simulink model "ZeroForceDrag_ThreeJoints"  (R2018b)
settings: Solver=FixedStepDiscrete  StartTime=0.0  StopTime=Inf  FixedStep=0.001  RelTol=1e-3  EnableMultiTasking=on
PreLoadFcn:
  | clear,clc;
undefined symbols (not defined in the file): J1, J2, J3, J4, J5, J6, J7, Motor_Current, Motor_Position, Motor_Velocity, Send_GUIdata
libraries: c280xlib x14, simulink x5, idelinklib_common x1
(part 4 of 4)

== stateflow chart ZeroForceDrag_ThreeJoints/DynamicCalculation/DriveMotor/驱动器指令/Chart2 ==
  state bx = check(write) [function]
  state MSG = UM1 [function]
  state start = start_arm(StartRobot) [function]
  state State05
    entry:
    start=0;
    during:
    start=start_arm(StartRobot);
    %启动机械臂
  state State01
    entry:
    bx=0;
    during:
    bx=check(write);
  state State06
    entry:
    MSG = UM1;
  state State03
    entry:
    MSG = BG;
  state MSG = TF(Current) [function]
  state State04
    entry:
    during:
    MSG = TF(Current);
  state MSG = BG [function]
  State01 -> State06 : [bx>0]
  (default) -> State05
  State05 -> State01 : [start>0]
  State06 -> State03
  State03 -> State04
  data: write function_input uint16 size=1; bx function_output uint16 size=1; MSG function_output; StartRobot function_input uint16 size=1; start function_output uint16 size=1; MSG function_output; Current function_input uint16 size=[1 6]; MSG function_output; MSG output; Current input size=[1 6]; write input uint16 size=1; bx local uint16 size=1; start local uint16; StartRobot input uint16
